simulink model "at40_pCtrl_q"  (R2016a)
settings: Solver=ode5  StartTime=0.0  StopTime=inf  FixedStep=0.001  RelTol=1e-3
undefined symbols (not defined in the file or in its folder): robot
libraries: simulink x9, dcpctrl x7
settings Model: SimulationMode=external  Creator=julianleland  LastModifiedBy=julianleland
settings HardwareCC: ProdBitPerLong=64  ProdLargestAtomicFloat=None  ProdHWDeviceType=Intel->x86-64  TargetBitPerLong=64  TargetBitPerPointer=64  TargetIntDivRoundTo=Zero  TargetEndianess=LittleEndian  TargetWordSize=64  TargetHWDeviceType=Intel->x86-64
settings RTWCC: SystemTargetFile=sldrt.tlc  TemplateMakefile=sldrt.tmf  Description=Simulink Desktop Real-Time  RTWCompilerOptimization=on
settings CodeAppCC: MaxIdLength=95
settings SimulinkDesktopRealTimeCC: TargetPreCompLibLocation=/Applications/MATLAB_R2016a.app/toolbox/sldrt/lib/maci64  TargetLangStandard=C89/C90 (ANSI)  SupportVariableSizeSignals=off

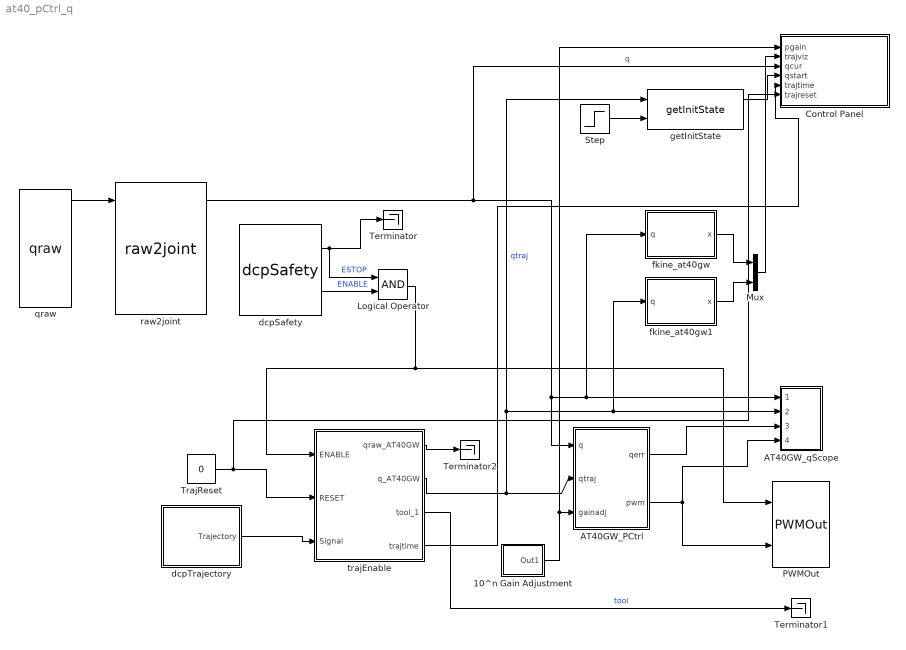
== system at40_pCtrl_q ==
  10^n Gain Adjustment : Subsystem
  AT40GW_PCtrl : Subsystem
  AT40GW_qScope : Subsystem
  Control Panel : Subsystem
  Logical Operator : Logic  AllPortsSameDT=off  OutDataTypeStr=boolean
  Mux : Mux  Inputs=2
  PWMOut : dcpctrl/PWMOut
  Step : Step  Time=0  SampleTime=0
  Terminator : Terminator
  Terminator1 : Terminator
  Terminator2 : Terminator
  TrajReset : Constant  Value=0
  dcpSafety : dcpctrl/dcpSafety
  dcpTrajectory : Subsystem
  fkine_at40gw : MATLAB Function  TreatAsAtomicUnit=on
  fkine_at40gw1 : MATLAB Function  TreatAsAtomicUnit=on
  getInitState : dcpctrl/getInitState
  qraw : dcpctrl/qraw
  raw2joint : dcpctrl/raw2joint
  trajEnable : Subsystem  AncestorBlock=dcpctrl/trajEnable
  wires:
  trajEnable/2(q_AT40GW) -> getInitState/1, fkine_at40gw1/1(q), AT40GW_qScope/2(Signal2), AT40GW_PCtrl/2(qtraj)  "qtraj"
  AT40GW_PCtrl/2(pwm) -> PWMOut/2, AT40GW_qScope/4(Signal4)
  AT40GW_PCtrl/1(qerr) -> AT40GW_qScope/3(Signal3)
  10^n Gain Adjustment/1(Out1) -> Control Panel/1(pgain), AT40GW_PCtrl/3("gainadj ")
  Logical Operator/1 -> trajEnable/1(ENABLE), PWMOut/1
  dcpSafety/1 -> Logical Operator/1, Terminator/1  "ESTOP"
  dcpSafety/2 -> Logical Operator/2  "ENABLE"
  trajEnable/3(tool_1) -> Terminator1/1  "tool"
  trajEnable/1(qraw_AT40GW) -> Terminator2/1
  qraw/1 -> raw2joint/1
  raw2joint/1 -> Control Panel/3(qcur), fkine_at40gw/1(q), AT40GW_qScope/1(Signal1), AT40GW_PCtrl/1(q)  "q"
  dcpTrajectory/1(Trajectory) -> trajEnable/3(Signal)
  fkine_at40gw/1(x) -> Mux/1
  Mux/1 -> Control Panel/2(trajviz)
  fkine_at40gw1/1(x) -> Mux/2
  TrajReset/1 -> Control Panel/6(trajreset), trajEnable/2(RESET)
  getInitState/1 -> Control Panel/4(qstart)
  Step/1 -> getInitState/2
  trajEnable/4(trajtime) -> Control Panel/5(trajtime)

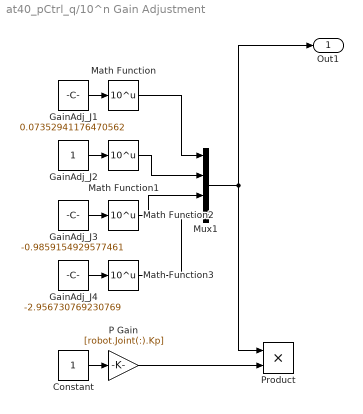
== system at40_pCtrl_q/10^n Gain Adjustment ==
  Constant : Constant
  GainAdj_J1 : Constant  Value=0.07352941176470562
  GainAdj_J2 : Constant
  GainAdj_J3 : Constant  Value=-0.9859154929577461
  GainAdj_J4 : Constant  Value=-2.956730769230769
  Math Function{,1..3} (4 alike) : Math  Operator=10^u  SaturateOnIntegerOverflow=on
  Mux1 : Mux
  P Gain : Gain  Gain=[robot.Joint(:).Kp]
  Product : Product
  Out1 : Outport
  wires:
  Math Function1/1 -> Mux1/2
  Math Function/1 -> Mux1/1
  Mux1/1 -> Out1/1, Product/1
  Math Function3/1 -> Mux1/4
  Math Function2/1 -> Mux1/3
  GainAdj_J1/1 -> Math Function/1
  GainAdj_J2/1 -> Math Function1/1
  GainAdj_J3/1 -> Math Function2/1
  GainAdj_J4/1 -> Math Function3/1
  Constant/1 -> P Gain/1
  P Gain/1 -> Product/2

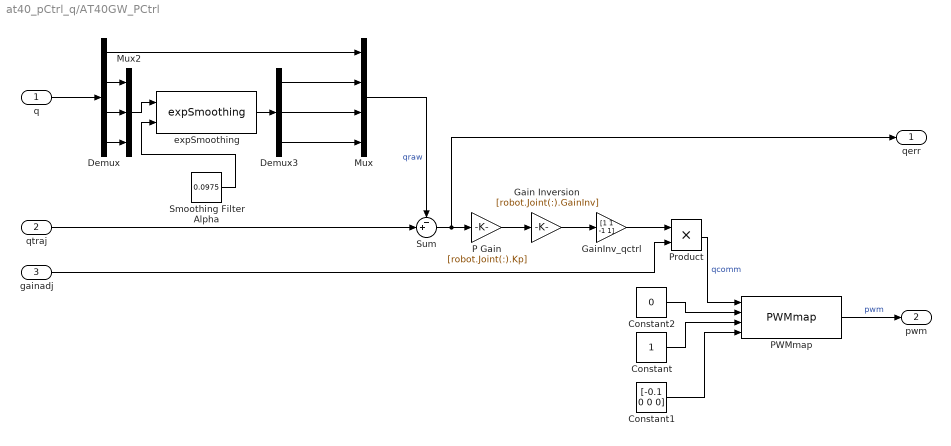
== system at40_pCtrl_q/AT40GW_PCtrl ==
  q : Inport
  qtraj : Inport  Port=2
  "gainadj " : Inport  Port=3
  Constant : Constant
  Constant1 : Constant  Value=[-0.1 0 0 0]
  Constant2 : Constant  Value=0
  Demux : Demux
  Demux3 : Demux  Outputs=3
  Gain Inversion : Gain  Gain=[robot.Joint(:).GainInv]
  GainInv_qctrl : Gain  Gain=[1 1 -1 1]
  Mux : Mux
  Mux2 : Mux  Inputs=3
  P Gain : Gain  Gain=[robot.Joint(:).Kp]
  PWMmap : dcpctrl/PWMmap
  Product : Product
  Smoothing Filter Alpha : Constant  Value=0.0975
  Sum : Sum  Inputs=-+|
  expSmoothing : dcpctrl/expSmoothing
  qerr : Outport
  pwm : Outport  Port=2
  wires:
  qtraj/1 -> Sum/2
  Mux/1 -> Sum/1  "qraw"
  Demux/1 -> Mux/1
  expSmoothing/1 -> Demux3/1
  Demux3/2 -> Mux/3
  Demux3/1 -> Mux/2
  Demux3/3 -> Mux/4
  Smoothing Filter Alpha/1 -> expSmoothing/2
  Mux2/1 -> expSmoothing/1
  Sum/1 -> qerr/1, P Gain/1
  PWMmap/1 -> pwm/1  "pwm"
  Product/1 -> PWMmap/1  "qcomm"
  P Gain/1 -> Gain Inversion/1
  "gainadj "/1 -> Product/2
  Gain Inversion/1 -> GainInv_qctrl/1
  Constant/1 -> PWMmap/3
  Constant1/1 -> PWMmap/4
  Constant2/1 -> PWMmap/2
  Demux/4 -> Mux2/3
  Demux/3 -> Mux2/2
  Demux/2 -> Mux2/1
  q/1 -> Demux/1
  GainInv_qctrl/1 -> Product/1

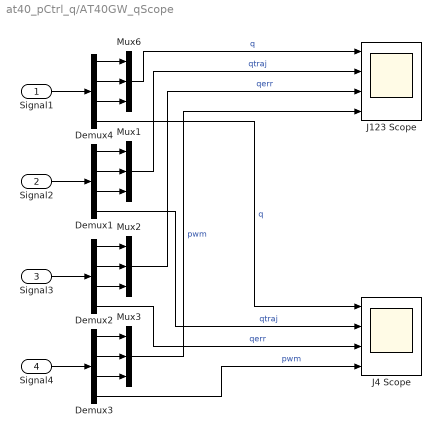
== system at40_pCtrl_q/AT40GW_qScope ==
  Signal1 : Inport
  Signal2 : Inport  Port=2
  Signal3 : Inport  Port=3
  Signal4 : Inport  Port=4
  Demux{1..4} (4 alike) : Demux
  J123 Scope : Scope  NumInputPorts=4
  J4 Scope : Scope  NumInputPorts=4
  Mux{1..3,6} (4 alike) : Mux  Inputs=3
  wires:
  Demux4/1 -> Mux6/1
  Mux3/1 -> J123 Scope/4  "pwm"
  Demux2/4 -> J4 Scope/3  "qerr"
  Demux1/4 -> J4 Scope/2  "qtraj"
  Mux6/1 -> J123 Scope/1  "q"
  Signal1/1 -> Demux4/1
  Demux4/2 -> Mux6/2
  Demux4/3 -> Mux6/3
  Demux1/1 -> Mux1/1
  Signal2/1 -> Demux1/1
  Demux1/2 -> Mux1/2
  Demux1/3 -> Mux1/3
  Demux2/1 -> Mux2/1
  Signal3/1 -> Demux2/1
  Demux2/2 -> Mux2/2
  Demux2/3 -> Mux2/3
  Demux3/1 -> Mux3/1
  Signal4/1 -> Demux3/1
  Demux3/2 -> Mux3/2
  Demux3/3 -> Mux3/3
  Mux1/1 -> J123 Scope/2  "qtraj"
  Mux2/1 -> J123 Scope/3  "qerr"
  Demux4/4 -> J4 Scope/1  "q"
  Demux3/4 -> J4 Scope/4  "pwm"

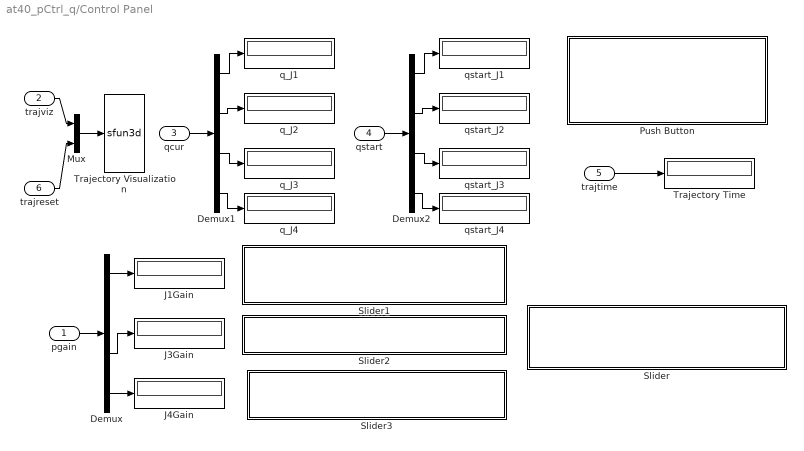
== system at40_pCtrl_q/Control Panel ==
  pgain : Inport
  trajviz : Inport  Port=2
  qcur : Inport  Port=3
  qstart : Inport  Port=4
  trajtime : Inport  Port=5
  trajreset : Inport  Port=6
  Demux : Demux
  Demux1 : Demux
  Demux2 : Demux
  J1Gain : Display
  J3Gain : Display
  J4Gain : Display
  Mux : Mux  Inputs=2
  Push Button : Subsystem  DialogController=hmiCreateDDGDialog  IsWebBlock=on  mask(MWDashboardBlock){webBlockId=d14440dc-dcfb-4a22-9820-9883405fda4f, webBlockType=pushbutton, ShowInLibBrwoser=on, ShowInitialText=on, HMISrcModelName=at40_pCtrl_qqd}
      mask prompts: webBlockId "WebBlock Id"; webBlockType "WebBlock Type"; HMISrcModelName "Source Model"
      mask Help: helpview([docroot '/mapfiles/simulink.map'], 'hmi_push_button')
      mask Display:
      | model = bdroot(gcb);
      | if strcmp(get_param(model,'BlockDiagramType'), 'library')
      |     image([(matlabroot) '/toolbox/simulink/hmi/icons/PushButton.png']);
      | end
  Slider : Subsystem  DialogController=hmiCreateDDGDialog  IsWebBlock=on  mask(MWDashboardBlock){webBlockId=f0c68e46-865a-4d96-89a7-5e1e8ebc446d, webBlockType=slider, ShowInLibBrowser=on, ShowInitialText=on, HMISrcModelName=at40_pCtrl_qqd}
      mask prompts: webBlockId "WebBlock Id"; webBlockType "WebBlock Type"; HMISrcModelName "Source Model"
      mask Help: helpview([docroot '/mapfiles/simulink.map'], 'hmi_slider')
      mask Display:
      | if strcmp(get_param(bdroot(gcb),'BlockDiagramType'), 'library')
      |     image([(matlabroot) '/toolbox/simulink/hmi/icons/Slider.png']);
      | end
  Slider1 : Subsystem  DialogController=hmiCreateDDGDialog  IsWebBlock=on  mask(MWDashboardBlock){webBlockId=1b4d9833-0382-4353-be8c-f20f38eb9aab, webBlockType=slider, ShowInLibBrowser=on, ShowInitialText=on, HMISrcModelName=at40_pCtrl_qqd}
      mask prompts: webBlockId "WebBlock Id"; webBlockType "WebBlock Type"; HMISrcModelName "Source Model"
      mask Help: helpview([docroot '/mapfiles/simulink.map'], 'hmi_slider')
      mask Display:
      | if strcmp(get_param(bdroot(gcb),'BlockDiagramType'), 'library')
      |     image([(matlabroot) '/toolbox/simulink/hmi/icons/Slider.png']);
      | end
  Slider2 : Subsystem  DialogController=hmiCreateDDGDialog  IsWebBlock=on  mask(MWDashboardBlock){webBlockId=cbf9babb-b489-42eb-b20a-0d2a912eb983, webBlockType=slider, ShowInLibBrowser=on, ShowInitialText=on, HMISrcModelName=at40_pCtrl_qqd}
      mask prompts: webBlockId "WebBlock Id"; webBlockType "WebBlock Type"; HMISrcModelName "Source Model"
      mask Help: helpview([docroot '/mapfiles/simulink.map'], 'hmi_slider')
      mask Display:
      | if strcmp(get_param(bdroot(gcb),'BlockDiagramType'), 'library')
      |     image([(matlabroot) '/toolbox/simulink/hmi/icons/Slider.png']);
      | end
  Slider3 : Subsystem  DialogController=hmiCreateDDGDialog  IsWebBlock=on  mask(MWDashboardBlock){webBlockId=af3345d3-46b3-4b00-a2f8-3f6dd7fd4884, webBlockType=slider, ShowInLibBrowser=on, ShowInitialText=on, HMISrcModelName=at40_pCtrl_qqd}
      mask prompts: webBlockId "WebBlock Id"; webBlockType "WebBlock Type"; HMISrcModelName "Source Model"
      mask Help: helpview([docroot '/mapfiles/simulink.map'], 'hmi_slider')
      mask Display:
      | if strcmp(get_param(bdroot(gcb),'BlockDiagramType'), 'library')
      |     image([(matlabroot) '/toolbox/simulink/hmi/icons/Slider.png']);
      | end
  Trajectory Time : Display
  Trajectory Visualization : S-Function  LoadFcn=if exist('sfun3d','file'), sfun3d([],[],[],'LoadBlock'); end  FunctionName=sfun3d  Parameters=ax,T,np,cp,gd,ls,mk  SFunctionDeploymentMode=off  EnableBusSupport=off  mask(3D Graph){np=2, ax=[2000 6000 -2000 2000 -2000 2000], cp=[6000 0 0 ], gd=on, ls=-, mk=., T=-1}
      mask prompts: np "Number of point (lines)"; ax "[xmin xmax  ymin ymax zmin zmax]"; cp "Camera position (use [0 0 1] for 2D XY view)"; gd "Grid (on|off)"; ls "LineStyle"; mk "Marker"; T "Sampling Time"
      mask help:
      | This block plots the position of several points in the XYZ space. The input contains the coordinates of all the points (x1,y1,z1,x2,y2,z2,...).
      | The number of points (lines), the XYZ ranges, camera position, grid, linestyle, marker and sampling time, can be set as mask parameters.
      settings: CopyFcn=if exist('sfun3d','file'), sfun3d([],[],[],'CopyBlock'); end  DeleteFcn=if exist('sfun3d','file'), sfun3d([],[],[],'DeleteBlock'); end  NameChangeFcn=if exist('sfun3d','file'), sfun3d([],[],[],'NameChange'); end
      mask Help:
      | This block plots the position of several points in the XYZ space. The input contains the coordinates of all the points (x1,y1,z1,x2,y2,z2,...).
      | The number of points (lines), the XYZ ranges, camera position, grid, linestyle, marker and sampling time, can be set as mask parameters.
      mask TypeOptions ls: - | -- | : | -. | none
      mask TypeOptions mk: none | . | + | o | * | x | square | diamond | v | ^ | > | < | pentagram | hexagram
      mask Display: plot([.05 .95 .95 .05 .05],[.45 .45 .95 .95 .45], 0.5+cos(0:0.1:2*pi)*0.3,0.7+sin(0:0.1:2*pi)*0.2)
  q_J{1..4} (4 alike) : Display
  qstart_J{1..4} (4 alike) : Display
  wires:
  pgain/1 -> Demux/1
  Demux/4 -> J4Gain/1
  Demux/1 -> J1Gain/1
  Demux/3 -> J3Gain/1
  trajviz/1 -> Mux/1
  qcur/1 -> Demux1/1
  Demux1/4 -> q_J4/1
  Demux1/1 -> q_J1/1
  Demux1/3 -> q_J3/1
  Demux1/2 -> q_J2/1
  qstart/1 -> Demux2/1
  Demux2/4 -> qstart_J4/1
  Demux2/1 -> qstart_J1/1
  Demux2/3 -> qstart_J3/1
  Demux2/2 -> qstart_J2/1
  trajtime/1 -> Trajectory Time/1
  trajreset/1 -> Mux/2
  Mux/1 -> Trajectory Visualization/1

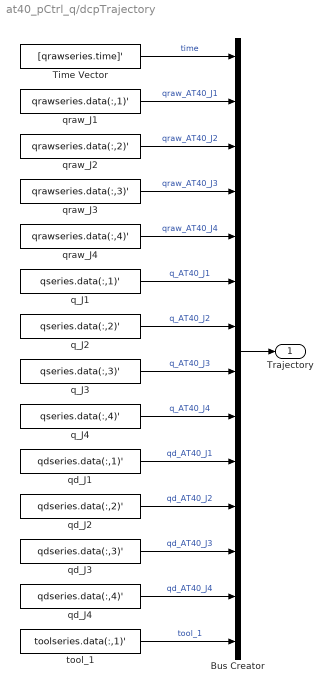
== system at40_pCtrl_q/dcpTrajectory ==
  Bus Creator : BusCreator  Inputs='time','qraw_AT40_J1','qraw_AT40_J2','qraw_AT40_J3','qraw_AT40_J4','q_AT40_J1','q_AT40_J2','q_AT40_J3','q_AT40_J4','qd_AT40_J1','qd_AT40_J2','qd_AT40_J3','qd_AT40_J4','tool_1'
  Time Vector : FromWorkspace  VariableName=[qrawseries.time]'  SampleTime=0
  q_J1 : FromWorkspace  VariableName=qseries.data(:,1)'  SampleTime=0
  q_J2 : FromWorkspace  VariableName=qseries.data(:,2)'  SampleTime=0
  q_J3 : FromWorkspace  VariableName=qseries.data(:,3)'  SampleTime=0
  q_J4 : FromWorkspace  VariableName=qseries.data(:,4)'  SampleTime=0
  qd_J1 : FromWorkspace  VariableName=qdseries.data(:,1)'  SampleTime=0
  qd_J2 : FromWorkspace  VariableName=qdseries.data(:,2)'  SampleTime=0
  qd_J3 : FromWorkspace  VariableName=qdseries.data(:,3)'  SampleTime=0
  qd_J4 : FromWorkspace  VariableName=qdseries.data(:,4)'  SampleTime=0
  qraw_J1 : FromWorkspace  VariableName=qrawseries.data(:,1)'  SampleTime=0
  qraw_J2 : FromWorkspace  VariableName=qrawseries.data(:,2)'  SampleTime=0
  qraw_J3 : FromWorkspace  VariableName=qrawseries.data(:,3)'  SampleTime=0
  qraw_J4 : FromWorkspace  VariableName=qrawseries.data(:,4)'  SampleTime=0
  tool_1 : FromWorkspace  VariableName=toolseries.data(:,1)'  SampleTime=0
  Trajectory : Outport
  wires:
  tool_1/1 -> Bus Creator/14  "tool_1"
  Bus Creator/1 -> Trajectory/1
  qraw_J4/1 -> Bus Creator/5  "qraw_AT40_J4"
  qraw_J2/1 -> Bus Creator/3  "qraw_AT40_J2"
  Time Vector/1 -> Bus Creator/1  "time"
  qraw_J3/1 -> Bus Creator/4  "qraw_AT40_J3"
  qraw_J1/1 -> Bus Creator/2  "qraw_AT40_J1"
  q_J1/1 -> Bus Creator/6  "q_AT40_J1"
  q_J2/1 -> Bus Creator/7  "q_AT40_J2"
  q_J3/1 -> Bus Creator/8  "q_AT40_J3"
  q_J4/1 -> Bus Creator/9  "q_AT40_J4"
  qd_J1/1 -> Bus Creator/10  "qd_AT40_J1"
  qd_J2/1 -> Bus Creator/11  "qd_AT40_J2"
  qd_J3/1 -> Bus Creator/12  "qd_AT40_J3"
  qd_J4/1 -> Bus Creator/13  "qd_AT40_J4"

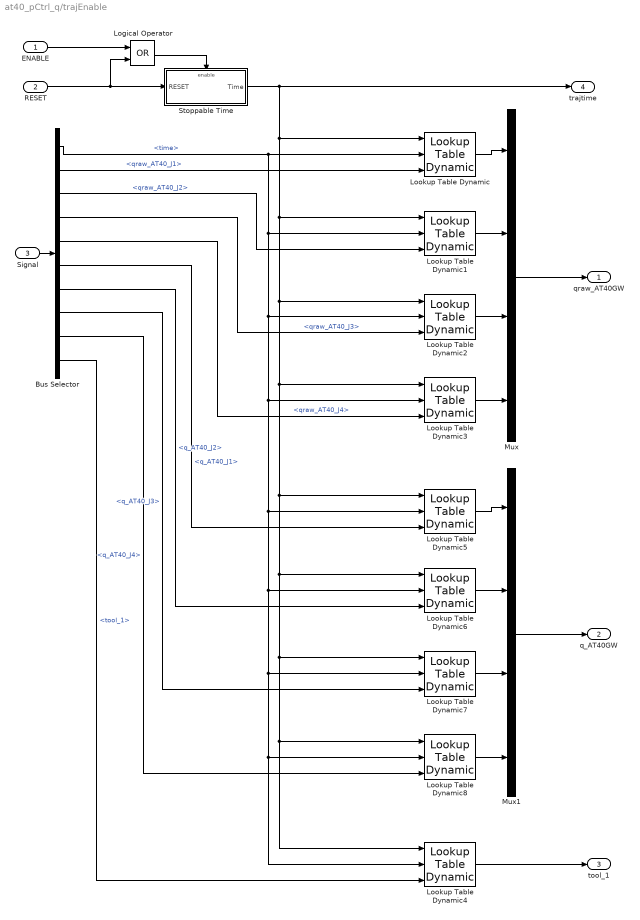
== system at40_pCtrl_q/trajEnable ==
  ENABLE : Inport
  RESET : Inport  Port=2
  Signal : Inport  Port=3
  Bus Selector : BusSelector  OutputSignals=time,qraw_AT40_J1,qraw_AT40_J2,qraw_AT40_J3,qraw_AT40_J4,q_AT40_J1,q_AT40_J2,q_AT40_J3,q_AT40_J4,tool_1
  Logical Operator : Logic  Operator=OR  AllPortsSameDT=off  OutDataTypeStr=boolean
  Lookup Table Dynamic{,1..8} (9 alike) : simulink/Lookup Tables/Lookup Table Dynamic  LookUpMeth=Interpolation-Use End Values  OutDataTypeStr=Inherit: Inherit via back propagation  OutDataType=fixdt('double')  OutScaling=2^-10  DoSatur=off
  Mux : Mux
  Mux1 : Mux
  Stoppable Time : Subsystem  TreatAsAtomicUnit=on
  qraw_AT40GW : Outport
  q_AT40GW : Outport  Port=2
  tool_1 : Outport  Port=3
  trajtime : Outport  Port=4
  wires:
  Bus Selector/5 -> Lookup Table Dynamic3/3  "<qraw_AT40_J4>"
  Lookup Table Dynamic/1 -> Mux/1
  Bus Selector/2 -> Lookup Table Dynamic/3  "<qraw_AT40_J1>"
  Bus Selector/3 -> Lookup Table Dynamic1/3  "<qraw_AT40_J2>"
  Bus Selector/4 -> Lookup Table Dynamic2/3  "<qraw_AT40_J3>"
  Lookup Table Dynamic3/1 -> Mux/4
  Lookup Table Dynamic2/1 -> Mux/3
  Lookup Table Dynamic1/1 -> Mux/2
  Mux/1 -> qraw_AT40GW/1
  Signal/1 -> Bus Selector/1
  Lookup Table Dynamic4/1 -> tool_1/1
  Bus Selector/10 -> Lookup Table Dynamic4/3  "<tool_1>"
  Stoppable Time/1(Time) -> trajtime/1, Lookup Table Dynamic5/1, Lookup Table Dynamic6/1, Lookup Table Dynamic7/1, Lookup Table Dynamic8/1, Lookup Table Dynamic4/1, Lookup Table Dynamic3/1, Lookup Table Dynamic2/1, Lookup Table Dynamic1/1, Lookup Table Dynamic/1
  Bus Selector/9 -> Lookup Table Dynamic8/3  "<q_AT40_J4>"
  Lookup Table Dynamic5/1 -> Mux1/1
  Bus Selector/6 -> Lookup Table Dynamic5/3  "<q_AT40_J1>"
  Bus Selector/7 -> Lookup Table Dynamic6/3  "<q_AT40_J2>"
  Bus Selector/1 -> Lookup Table Dynamic5/2, Lookup Table Dynamic7/2, Lookup Table Dynamic8/2, Lookup Table Dynamic4/2, Lookup Table Dynamic6/2, Lookup Table Dynamic3/2, Lookup Table Dynamic2/2, Lookup Table Dynamic1/2, Lookup Table Dynamic/2  "<time>"
  Bus Selector/8 -> Lookup Table Dynamic7/3  "<q_AT40_J3>"
  Lookup Table Dynamic8/1 -> Mux1/4
  Lookup Table Dynamic7/1 -> Mux1/3
  Lookup Table Dynamic6/1 -> Mux1/2
  Mux1/1 -> q_AT40GW/1
  RESET/1 -> Stoppable Time/1(RESET), Logical Operator/2
  ENABLE/1 -> Logical Operator/1
  Logical Operator/1 -> Stoppable Time/Enable

== system at40_pCtrl_q/Control Panel/Push Button ==

== system at40_pCtrl_q/Control Panel/Slider ==

== system at40_pCtrl_q/Control Panel/Slider1 ==

== system at40_pCtrl_q/Control Panel/Slider2 ==

== system at40_pCtrl_q/Control Panel/Slider3 ==

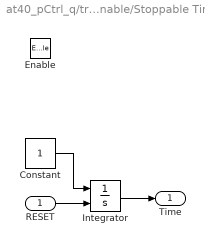
== system at40_pCtrl_q/trajEnable/Stoppable Time ==
  RESET : Inport
  Enable : EnablePort
  Constant : Constant
  Integrator : Integrator  ExternalReset=level hold
  Time : Outport
  wires:
  Constant/1 -> Integrator/1
  Integrator/1 -> Time/1
  RESET/1 -> Integrator/2

== matlab function at40_pCtrl_q/fkine_at40gw1 ==
  data: q input; x output
function x = fcn(q)
%#codegen

x_temp = fkine_at40gw(q(1),q(2),q(3),q(4))*[1;0;0;0];
x = x_temp(2:4);

== matlab function at40_pCtrl_q/fkine_at40gw ==
  data: q input; x output
function x = fcn(q)
%#codegen

x_temp = fkine_at40gw(q(1),q(2),q(3),q(4))*[1;0;0;0];
x = x_temp(2:4);
